simulink model "noise_tvg"  (R2012b)
settings: Solver=ode45  StartTime=0.0  StopTime=50000  RelTol=1e-3
libraries: xbsIndex_r4 x12, casper_library_sources x2
settings Model: Creator=paulp  LastModifiedBy=paulp

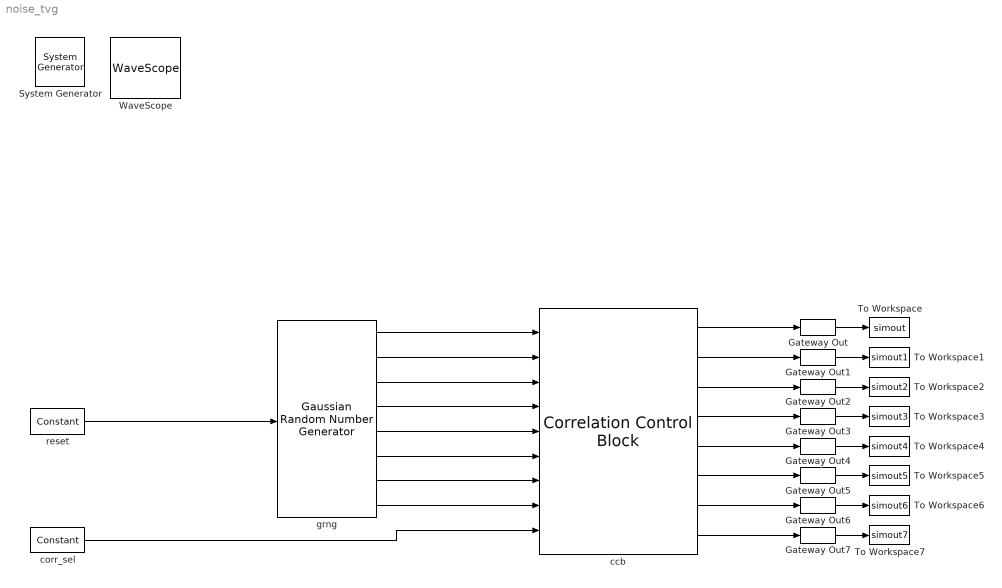
== system noise_tvg ==
  " System Generator" : xbsIndex_r4/ System Generator  Tag=genX  xilinxfamily=Kintex7  part=xc7k325t  speed=-3  package=fbg676  synthesis_tool=XST  clock_wrapper=Clock Enables  directory=./netlist  proj_type=Project Navigator  Synth_file=XST Defaults  Impl_file=ISE Defaults  testbench=off  simulink_period=1  sysclk_period=10  dcm_input_clock_period=10  incr_netlist=off  trim_vbits=Everywhere in SubSystem  dbl_ovrd=According to Block Masks  core_generation=According to Block Masks  run_coregen=off  deprecated_control=off  eval_field=0  block_type=sysgen
  Gateway Out{,1..7} (8 alike) : xbsIndex_r4/Gateway Out  inherit_from_input=off  hdl_port=off  timing_constraint=None  locs_specified=off  LOCs={}  UseAsDAC=off  DACChannel='1'  block_type=gatewayout
  To Workspace : ToWorkspace  VariableName=simout  SampleTime=-1  SaveFormat=Timeseries
  To Workspace1 : ToWorkspace  VariableName=simout1  SampleTime=-1  SaveFormat=Timeseries
  To Workspace2 : ToWorkspace  VariableName=simout2  SampleTime=-1  SaveFormat=Timeseries
  To Workspace3 : ToWorkspace  VariableName=simout3  SampleTime=-1  SaveFormat=Timeseries
  To Workspace4 : ToWorkspace  VariableName=simout4  SampleTime=-1  SaveFormat=Timeseries
  To Workspace5 : ToWorkspace  VariableName=simout5  SampleTime=-1  SaveFormat=Timeseries
  To Workspace6 : ToWorkspace  VariableName=simout6  SampleTime=-1  SaveFormat=Timeseries
  To Workspace7 : ToWorkspace  VariableName=simout7  SampleTime=-1  SaveFormat=Timeseries
  WaveScope : xbsIndex_r4/WaveScope  block_type=wavescope
  ccb : casper_library_sources/Correlation Control Block
  corr_sel : xbsIndex_r4/Constant  const=0  gui_display_data_type=Fixed-point  arith_type=Unsigned  n_bits=3  bin_pt=0  preci_type=Single  exp_width=8  frac_width=24  explicit_period=on  period=1  equ=P=C  opselect=C  inp2=PCIN>>17  opr=+  inp1=P  carry=CIN  dbl_ovrd=off  block_type=constant
  grng : casper_library_sources/Gaussian Random Number Generator
  reset : xbsIndex_r4/Constant  const=0  gui_display_data_type=Boolean  arith_type=Boolean  n_bits=16  bin_pt=14  preci_type=Single  exp_width=8  frac_width=24  explicit_period=on  period=1  equ=P=C  opselect=C  inp2=PCIN>>17  opr=+  inp1=P  carry=CIN  dbl_ovrd=off  block_type=constant
  wires:
  grng/5 -> ccb/5
  grng/4 -> ccb/4
  grng/6 -> ccb/6
  grng/3 -> ccb/3
  grng/2 -> ccb/2
  grng/7 -> ccb/7
  grng/1 -> ccb/1
  grng/8 -> ccb/8
  reset/1 -> grng/1
  corr_sel/1 -> ccb/9
  ccb/1 -> Gateway Out/1
  ccb/2 -> Gateway Out1/1
  ccb/3 -> Gateway Out2/1
  ccb/4 -> Gateway Out3/1
  ccb/5 -> Gateway Out4/1
  ccb/6 -> Gateway Out5/1
  ccb/7 -> Gateway Out6/1
  ccb/8 -> Gateway Out7/1
  Gateway Out/1 -> To Workspace/1
  Gateway Out1/1 -> To Workspace1/1
  Gateway Out3/1 -> To Workspace3/1
  Gateway Out4/1 -> To Workspace4/1
  Gateway Out5/1 -> To Workspace5/1
  Gateway Out6/1 -> To Workspace6/1
  Gateway Out7/1 -> To Workspace7/1
  Gateway Out2/1 -> To Workspace2/1
